simulink model "spiBitbangSimulink_v2"  (R2013b)
settings: Solver=FixedStepDiscrete  StartTime=0.0  StopTime=5e-3  FixedStep=sampleTime  MaxStep=MaxStepSize  RelTol=1e-3
undefined symbols (not defined in the file or in its folder): sampleTime
libraries: simulink x1, dspswit3 x1, simulink_extras x1
settings Model: ExtModeTrigDuration=100  Creator=mainster  LastModifiedBy=mainster
settings OptimizationCC: OptimizeModelRefInitCode=on  LifeSpan=1
settings DebuggingCC: SolverPrmCheckMsg=none
settings HardwareCC: ProdLargestAtomicInteger=Long  ProdLargestAtomicFloat=Double  ProdEndianess=LittleEndian  ProdHWDeviceType=ARM Compatible->ARM Cortex
settings RTWCC: SystemTargetFile=realtime.tlc  GenerateMakefile=off  TemplateMakefile=realtime.tmf  Description=Run on Target Hardware  RTWVerbose=off  ProcessScript=realtime_make_rtw_hook
settings STFCustomTargetCC: TargetLibSuffix=.a  GenerateSampleERTMain=on  ERTCustomFileBanners=on  SupportNonInlinedSFcns=off  SupportVariableSizeSignals=on  MATLABClassNameForMDSCustomization=Simulink.SoftwareTarget.ERTCustomization  GRTInterface=off  SystemTargetFile=realtime.tlc
settings ERTTargetCC: CodeReplacementLibrary=ANSI_C  GenerateSampleERTMain=on  ParMdlRefBuildCompliant=off  CompOptLevelCompliant=off  ConcurrentExecutionCompliant=off  CombineOutputUpdateFcns=off  ERTFirstTimeCompliant=off  SupportContinuousTime=on  SupportVariableSizeSignals=on  ModelStepFunctionPrototypeControlCompliant=off  CPPClassGenCompliant=off  ExtModeMexArgs='192.168.2.111' 0 17725  InlinedParameterPlacement=NonHierarchical  ERTSrcFileBannerTemplate=realtime_code_template.cgt  ERTHdrFileBannerTemplate=realtime_code_template.cgt  ERTDataSrcFileTemplate=realtime_code_template.cgt  ERTDataHdrFileTemplate=realtime_code_template.cgt  ERTCustomFileTemplate=realtime_file_process.tlc

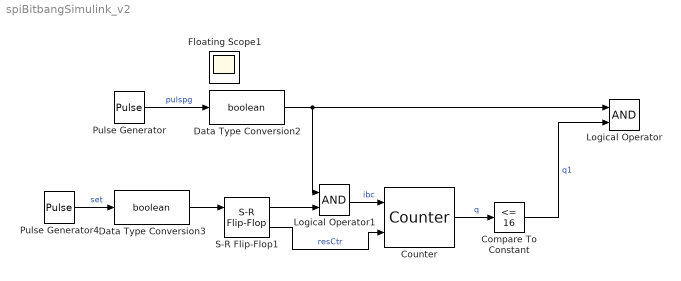
== system spiBitbangSimulink_v2 ==
  Compare To Constant : simulink/Logic and Bit Operations/Compare To Constant  relop=<=  const=16  OutDataTypeStr=boolean
  Counter : dspswit3/Counter  Direction=Up  CountEvent=Rising edge  CounterSize=8 bits  MaxCount=255  InitialCount=0  Output=Count  HitValue=32  ResetInput=on  SamplesPerFrame=1  Ts=1  CntDtype=uint8  HitDtype=Logical
  Data Type Conversion2 : DataTypeConversion  OutDataTypeStr=boolean
  Data Type Conversion3 : DataTypeConversion  OutDataTypeStr=boolean
  Logical Operator : Logic  AllPortsSameDT=off  OutDataTypeStr=boolean
  Logical Operator1 : Logic  AllPortsSameDT=off  OutDataTypeStr=boolean
  Pulse Generator : DiscretePulseGenerator  Period=83  PulseWidth=25  SampleTime=sampleTime
  Pulse Generator4 : DiscretePulseGenerator  Period=100  PulseWidth=50  PhaseDelay=10  SampleTime=sampleTime
  S-R Flip-Flop1 : simulink_extras/Flip Flops/S-R Flip-Flop  initial_condition=0
  Floating Scope1 : Scope
      settings: Floating=on  SaveName=ScopeData3
  wires:
  Pulse Generator/1 -> Data Type Conversion2/1  "pulspg"
  Counter/1 -> Compare To Constant/1  "q"
  Compare To Constant/1 -> Logical Operator/2  "q1"
  S-R Flip-Flop1/1 -> Logical Operator1/2
  Logical Operator1/1 -> Counter/1  "ibc"
  Pulse Generator4/1 -> Data Type Conversion3/1  "set"
  S-R Flip-Flop1/2 -> Counter/2  "resCtr"
  Data Type Conversion2/1 -> Logical Operator1/1, Logical Operator/1
  Data Type Conversion3/1 -> S-R Flip-Flop1/1
